simulink model "Fig423"  (R2014b)
settings: Solver=ode3  StartTime=0.0  StopTime=5.24288  FixedStep=2e-5  RelTol=1e-3
libraries: simulink_extras x1, commrandsrc2 x1
settings Model: Creator=Dennis Silage  LastModifiedBy=Silage
settings DataIOCC: SignalLoggingSaveFormat=ModelDataLogs
settings OptimizationCC: ExpressionDepthLimit=2147483647  InitFltsAndDblsToZero=on
settings DebuggingCC: UnderspecifiedInitializationDetection=Classic  MergeDetectMultiDrivingBlocksExec=none  FcnCallInpInsideContextMsg=UseLocalSettings  StateNameClashWarn=warning  StrictBusMsg=Warning
settings GRTTargetCC: CombineOutputUpdateFcns=off  GRTInterface=on

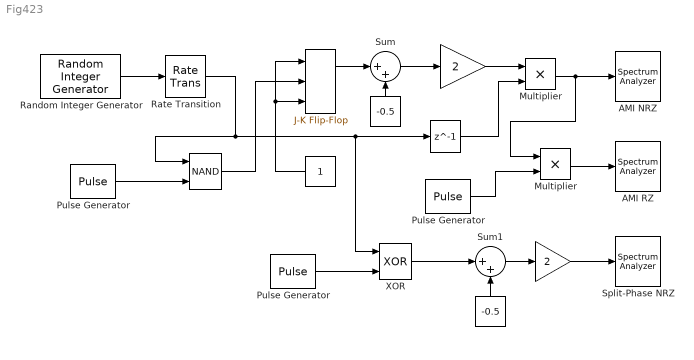
== system Fig423 ==
  " " : Constant  Value=-0.5
  "   " : Gain  Gain=2
  "     " : Delay  DelayLength=1  InputProcessing=Inherited
  "      " : Gain  Gain=2
  "       " : simulink_extras/Flip Flops/J-K Flip-Flop  initial_condition=0
  "        " : Logic  Operator=NAND  IconShape=distinctive  AllPortsSameDT=off  OutDataTypeStr=boolean
  "             " : Constant  Value=-0.5
  "              " : Constant  OutDataTypeStr=boolean
  AMI NRZ : SpectrumAnalyzer
  AMI RZ : SpectrumAnalyzer
  Multiplier : Product  RndMeth=Zero
  "Multiplier " : Product  RndMeth=Zero
  "Pulse Generator " : DiscretePulseGenerator  Period=50  PulseWidth=25  SampleTime=2e-5
  "Pulse Generator  " : DiscretePulseGenerator  Period=50  PhaseDelay=1  SampleTime=2e-5
  Pulse Generator : DiscretePulseGenerator  Period=50  PulseWidth=25  PhaseDelay=1  SampleTime=2e-5
  Random Integer Generator : commrandsrc2/Random Integer Generator  mul=2  seed=randseed  Ts=1e-3  frameBased=off  sampPerFrame=1  orient=off  outDataType=double
  Rate Transition : RateTransition
  Split-Phase NRZ : SpectrumAnalyzer
  Sum : Sum  Inputs=|++
  Sum1 : Sum  Inputs=|++
  XOR : Logic  Operator=XOR  IconShape=distinctive  AllPortsSameDT=off  OutDataTypeStr=boolean
  wires:
  Sum/1 -> "   "/1
  " "/1 -> Sum/2
  "Pulse Generator  "/1 -> "        "/2
  Random Integer Generator/1 -> Rate Transition/1
  "       "/1 -> Sum/1
  Rate Transition/1 -> "        "/1, XOR/1, "     "/1
  "   "/1 -> Multiplier/1
  Multiplier/1 -> "Multiplier "/1, AMI NRZ/1
  "     "/1 -> Multiplier/2
  "Multiplier "/1 -> AMI RZ/1
  "Pulse Generator "/1 -> XOR/2
  "              "/1 -> "       "/1, "       "/3
  "        "/1 -> "       "/2
  "      "/1 -> Split-Phase NRZ/1
  "             "/1 -> Sum1/2
  XOR/1 -> Sum1/1
  Sum1/1 -> "      "/1
  Pulse Generator/1 -> "Multiplier "/2
